simulink model "ControlVehiculoV_ACT"  (R2023b)
settings: Solver=VariableStepAuto  StartTime=0.0  StopTime=10.0  RelTol=1e-3
model workspace (MAT data in the model file):
  d = 0.21
settings Model: Creator=Alberto  LastModifiedBy=Alberto

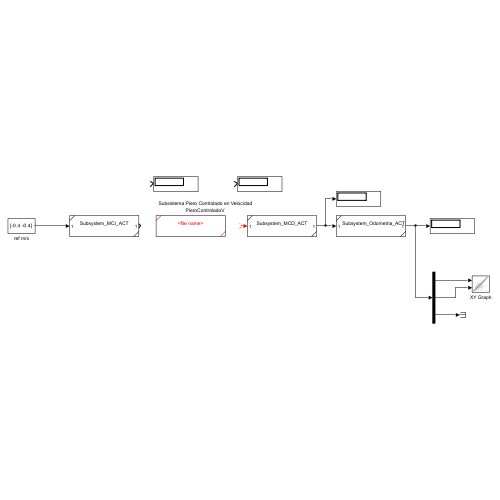
[thumbnail: Simulink's stored preview of the top-level diagram]
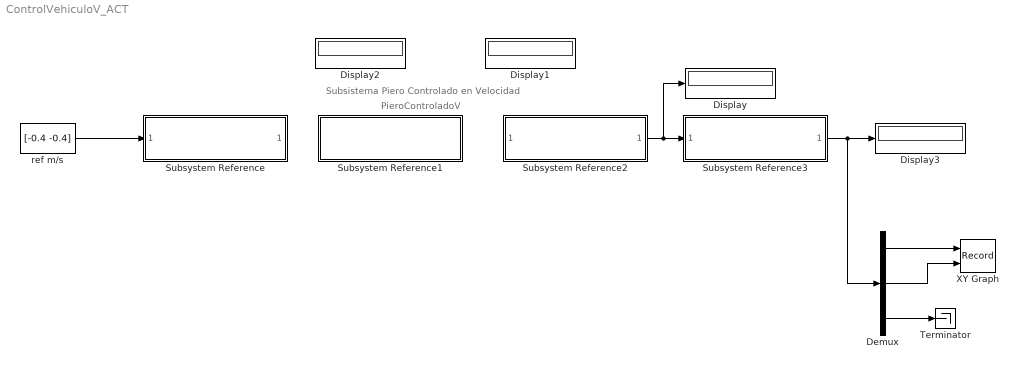
== system ControlVehiculoV_ACT ==
  note: PieroControladoV
  note: Subsistema Piero Controlado en Velocidad
  Demux : Demux  Outputs=3
  Display{,1..3} (4 alike) : Display
  Subsystem Reference : Subsystem  ReferencedSubsystem=Subsystem_MCI_ACT
  Subsystem Reference1 : Subsystem  ReferencedSubsystem=<file name>
  Subsystem Reference2 : Subsystem  ReferencedSubsystem=Subsystem_MCD_ACT
  Subsystem Reference3 : Subsystem  ReferencedSubsystem=Subsystem_Odometria_ACT
  Terminator : Terminator
  XY Graph : Record  FileSettingsInternal="{\"entries\":[{\"content\":{\"excelSettings\":{\"content\":{},\"type\":\"Streamout.ExcelSettings\"}},\"type\":\"Streamout.FileSettingStorage\",\"uuid\":\"\"}],\"packageUris\":[\"http:\\/\\/schema.mathworks.com\\/mf0\\/streamout_blocks\\/R2020a\"],\"version\":\"1.0\"}"  Layout=[1 1]  SignalsInternal="{\"entries\":[{\"content\":{\"signals\":[{\"content\":{\"blockPath\":[],\"dimensions\":[1],\"domain\":\"\",\"lineColor\":\"#a2142f\",\"plots\":[ 1 ],\"port\":1,\"signalID\":1,\"signalName\":\"XY Graph:1\"},\"type\":\"RecordBlkView.Signal\",\"uuid\":\"\"},{\"content\":{\"blockPath\":[],\"dimensions\":[1],\"domain\":\"\",\"lineColor\":\"#139fff\",\"plots\":[ 1 ],\"port\":2,\"signalID\":2,\"signalName\":\"XY Graph:2\"},\"type\":\"RecordBlkView.Signal\",\"uuid\":\"\"}]},\"type\":\"RecordBlkView.InputSignals\",\"uuid\":\"\"}],\"packageUris\":[\"http:\\/\\/schema.mathworks.com\\/mf0\\/streamout_blocks\\/R2020a\"],\"version\":\"1.0\"}"  VisualizationBindings="{\"xyplotplugin\":{\"info\":[{\"series\":[{\"bindingParametersList\":[{\"parameter\":\"X-Axis\",\"signalID\":1,\"signalName\":\"XY Graph:1\"},{\"parameter\":\"Y-Axis\",\"signalID\":2,\"signalName\":\"XY Graph:2\"}],\"seriesID\":0}],\"subplotID\":1}]}}"  CompatibilityTag=XY
  ref m/s : Constant  Value=[-0.4 -0.4]
  wires:
  Subsystem Reference2/1 -> Display/1, Subsystem Reference3/1
  ref m/s/1 -> Subsystem Reference/1
  ? -> Subsystem Reference2/1
  Subsystem Reference3/1 -> Demux/1, Display3/1
  Demux/1 -> XY Graph/1
  Demux/2 -> XY Graph/2
  Demux/3 -> Terminator/1

== system ControlVehiculoV_ACT/Subsystem Reference1 ==
